simulink model "vehicle_model10DOF"  (R2020a)
settings: Solver=VariableStepAuto  StartTime=0.0  StopTime=10.0  RelTol=1e-3
values from neighbouring files (symbols this model uses):
  a = 1.05    [model_init.m]
  b = 1.8-a    (= 0.75)    [model_init.m]
  Bd = 0.1    [model_init.m]
  c = 1.5    [model_init.m]
  I = m*a*b    (= 1496.25)    [model_init.m]
  Idf = 0.805    [model_init.m]
  Idr = 0.805    [model_init.m]
  m = 1900    [model_init.m]
  r = 0.3284    [model_init.m]
undefined symbols (not defined in the file or in its folder): psi0, psidot0, vw, wfl0, wfr0, wrl0, wrr0, X0, xdot0, Y0, ydot0
settings Model: Creator=Ivona  LastModifiedBy=Ivona

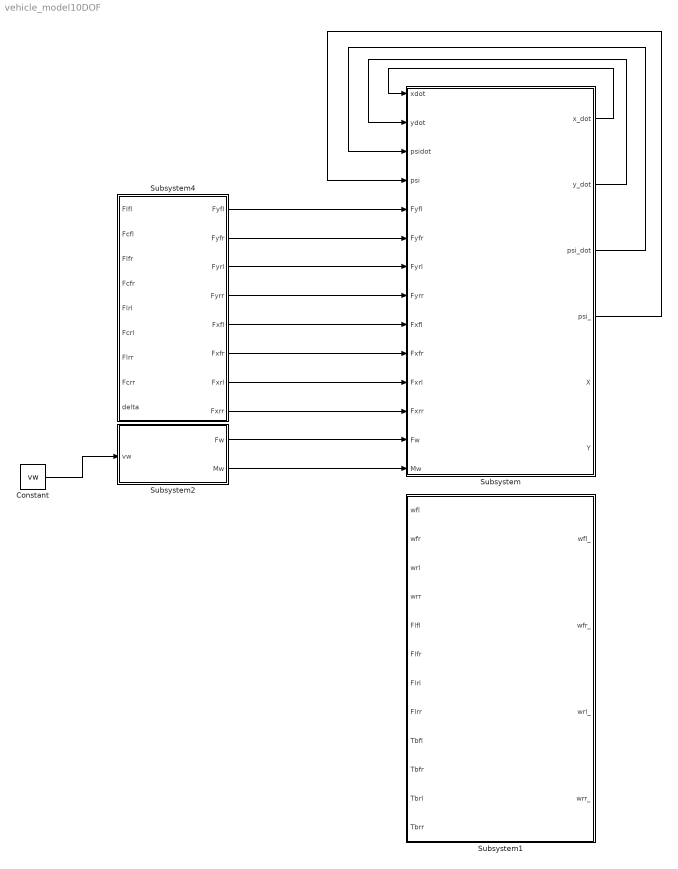
== system vehicle_model10DOF ==
  Constant : Constant  Value=vw
  Subsystem : Subsystem
  Subsystem1 : Subsystem
  Subsystem2 : Subsystem
  Subsystem4 : Subsystem
  wires:
  Subsystem/4(psi_) -> Subsystem/4(psi)
  Constant/1 -> Subsystem2/1(vw)
  Subsystem/3(psi_dot) -> Subsystem/3(psidot)
  Subsystem/2(y_dot) -> Subsystem/2(ydot)
  Subsystem4/3(Fyrl) -> Subsystem/7(Fyrl)
  Subsystem4/7(Fxrl) -> Subsystem/11(Fxrl)
  Subsystem/1(x_dot) -> Subsystem/1(xdot)
  Subsystem4/6(Fxfr) -> Subsystem/10(Fxfr)
  Subsystem4/5(Fxfl) -> Subsystem/9(Fxfl)
  Subsystem2/2(Mw) -> Subsystem/14(Mw)
  Subsystem2/1(Fw) -> Subsystem/13(Fw)
  Subsystem4/1(Fyfl) -> Subsystem/5(Fyfl)
  Subsystem4/4(Fyrr) -> Subsystem/8(Fyrr)
  Subsystem4/2(Fyfr) -> Subsystem/6(Fyfr)
  Subsystem4/8(Fxrr) -> Subsystem/12(Fxrr)

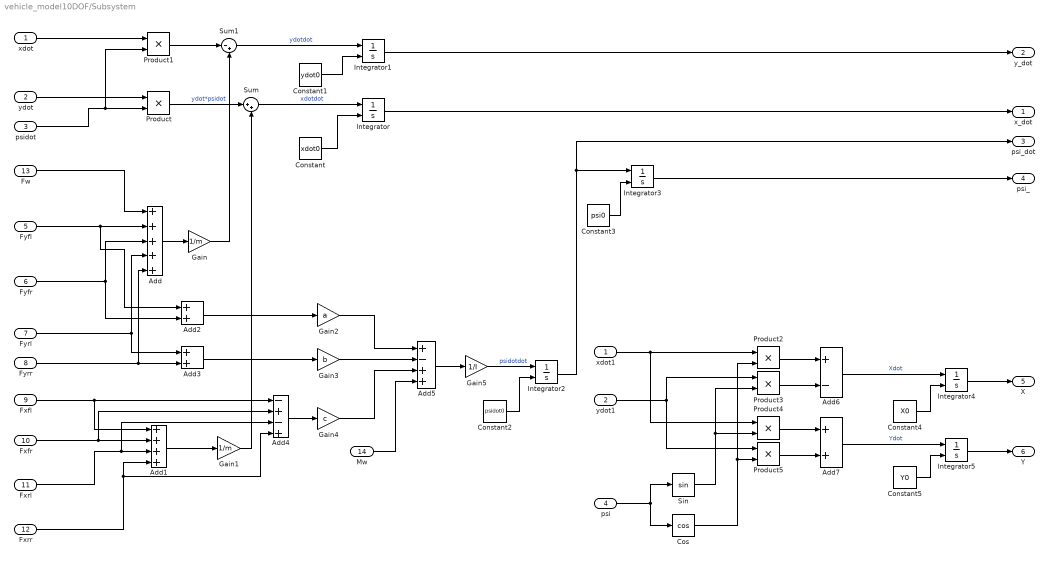
== system vehicle_model10DOF/Subsystem ==
  xdot : Inport
  ydot : Inport  Port=2
  psidot : Inport  Port=3
  psi : Inport  Port=4
  Fyfl : Inport  Port=5
  Fyfr : Inport  Port=6
  Fyrl : Inport  Port=7
  Fyrr : Inport  Port=8
  Fxfl : Inport  Port=9
  Fxfr : Inport  Port=10
  Fxrl : Inport  Port=11
  Fxrr : Inport  Port=12
  Fw : Inport  Port=13
  Mw : Inport  Port=14
  Add : Sum  Inputs=+++++
  Add1 : Sum  Inputs=++++
  Add2 : Sum
  Add3 : Sum
  Add4 : Sum  Inputs=-+-+
  Add5 : Sum  Inputs=+-++
  Add6 : Sum  Inputs=+-
  Add7 : Sum
  Constant : Constant  Value=xdot0
  Constant1 : Constant  Value=ydot0
  Constant2 : Constant  Value=psidot0
  Constant3 : Constant  Value=psi0
  Constant4 : Constant  Value=X0
  Constant5 : Constant  Value=Y0
  Cos : Trigonometry  Operator=cos
  Gain : Gain  Gain=1/m
  Gain1 : Gain  Gain=1/m
  Gain2 : Gain  Gain=a
  Gain3 : Gain  Gain=b
  Gain4 : Gain  Gain=c
  Gain5 : Gain  Gain=1/I
  Integrator{,1..5} (6 alike) : Integrator  InitialConditionSource=external
  Product{,1..5} (6 alike) : Product
  Sin : Trigonometry
  Sum : Sum  Inputs=|++
  Sum1 : Sum  Inputs=|-+
  xdot1 : InportShadow
  ydot1 : InportShadow  Port=2
  x_dot : Outport
  y_dot : Outport  Port=2
  psi_dot : Outport  Port=3
  psi_ : Outport  Port=4
  X : Outport  Port=5
  Y : Outport  Port=6
  wires:
  ydot/1 -> Product/1
  psidot/1 -> Product1/2, Product/2
  Fyfl/1 -> Add/2, Add2/1
  Fyfr/1 -> Add/3, Add2/2
  Fyrl/1 -> Add3/1, Add/4
  Fyrr/1 -> Add/5, Add3/2
  Add/1 -> Gain/1
  Product/1 -> Sum/1  "ydot*psidot"
  Sum/1 -> Integrator/1  "xdotdot"
  Constant/1 -> Integrator/2
  Integrator/1 -> x_dot/1
  xdot/1 -> Product1/1
  Product1/1 -> Sum1/1
  Fxfl/1 -> Add1/1, Add4/1
  Fxfr/1 -> Add4/2, Add1/2
  Fxrl/1 -> Add4/3, Add1/3
  Fxrr/1 -> Add4/4, Add1/4
  Add1/1 -> Gain1/1
  Sum1/1 -> Integrator1/1  "ydotdot"
  Constant1/1 -> Integrator1/2
  Integrator1/1 -> y_dot/1
  Add2/1 -> Gain2/1
  Add3/1 -> Gain3/1
  Add4/1 -> Gain4/1
  Gain2/1 -> Add5/1
  Gain3/1 -> Add5/2
  Gain4/1 -> Add5/3
  Add5/1 -> Gain5/1
  Gain5/1 -> Integrator2/1  "psidotdot"
  Constant2/1 -> Integrator2/2
  Integrator2/1 -> Integrator3/1, psi_dot/1
  Integrator3/1 -> psi_/1
  Constant3/1 -> Integrator3/2
  psi/1 -> Sin/1, Cos/1
  Product2/1 -> Add6/1
  Product3/1 -> Add6/2
  xdot1/1 -> Product4/1, Product2/1
  Cos/1 -> Product5/2, Product2/2
  ydot1/1 -> Product5/1, Product3/1
  Sin/1 -> Product4/2, Product3/2
  Product4/1 -> Add7/1
  Product5/1 -> Add7/2
  Add6/1 -> Integrator4/1  "Xdot"
  Integrator4/1 -> X/1
  Constant4/1 -> Integrator4/2
  Add7/1 -> Integrator5/1  "Ydot"
  Integrator5/1 -> Y/1
  Constant5/1 -> Integrator5/2
  Gain/1 -> Sum1/2
  Gain1/1 -> Sum/2
  Fw/1 -> Add/1
  Mw/1 -> Add5/4

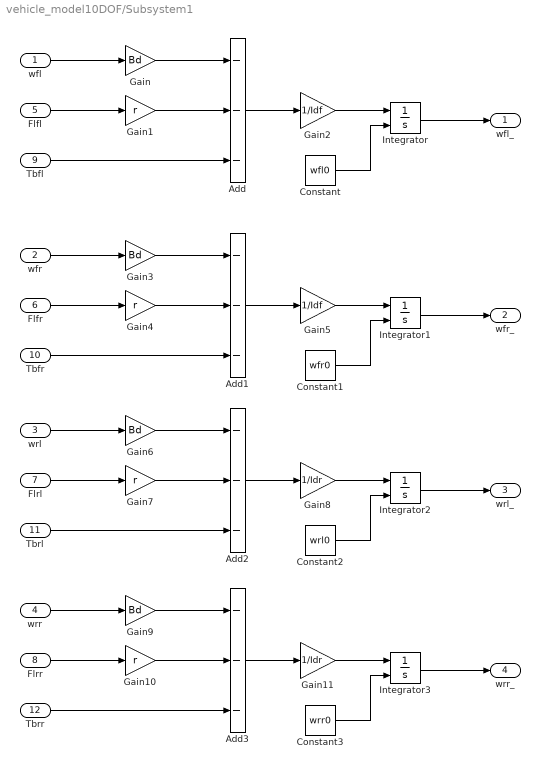
== system vehicle_model10DOF/Subsystem1 ==
  wfl : Inport
  wfr : Inport  Port=2
  wrl : Inport  Port=3
  wrr : Inport  Port=4
  Flfl : Inport  Port=5
  Flfr : Inport  Port=6
  Flrl : Inport  Port=7
  Flrr : Inport  Port=8
  Tbfl : Inport  Port=9
  Tbfr : Inport  Port=10
  Tbrl : Inport  Port=11
  Tbrr : Inport  Port=12
  Add{,1..3} (4 alike) : Sum  Inputs=---
  Constant : Constant  Value=wfl0
  Constant1 : Constant  Value=wfr0
  Constant2 : Constant  Value=wrl0
  Constant3 : Constant  Value=wrr0
  Gain{,3,6,9} (4 alike) : Gain  Gain=Bd
  Gain{1,4,7,10} (4 alike) : Gain  Gain=r
  Gain11 : Gain  Gain=1/Idr
  Gain2 : Gain  Gain=1/Idf
  Gain5 : Gain  Gain=1/Idf
  Gain8 : Gain  Gain=1/Idr
  Integrator{,1..3} (4 alike) : Integrator  InitialConditionSource=external
  wfl_ : Outport
  wfr_ : Outport  Port=2
  wrl_ : Outport  Port=3
  wrr_ : Outport  Port=4
  wires:
  Gain/1 -> Add/1
  Tbfl/1 -> Add/3
  Flfl/1 -> Gain1/1
  wfl/1 -> Gain/1
  Gain1/1 -> Add/2
  Add/1 -> Gain2/1
  Gain2/1 -> Integrator/1
  Constant/1 -> Integrator/2
  Integrator/1 -> wfl_/1
  Tbfr/1 -> Add1/3
  wfr/1 -> Gain3/1
  Gain3/1 -> Add1/1
  Flfr/1 -> Gain4/1
  Gain4/1 -> Add1/2
  Add1/1 -> Gain5/1
  Integrator1/1 -> wfr_/1
  Gain5/1 -> Integrator1/1
  Constant1/1 -> Integrator1/2
  Gain8/1 -> Integrator2/1
  Add2/1 -> Gain8/1
  Tbrl/1 -> Add2/3
  wrl/1 -> Gain6/1
  Constant2/1 -> Integrator2/2
  Integrator2/1 -> wrl_/1
  Gain7/1 -> Add2/2
  Gain6/1 -> Add2/1
  Flrl/1 -> Gain7/1
  Gain11/1 -> Integrator3/1
  Add3/1 -> Gain11/1
  Tbrr/1 -> Add3/3
  wrr/1 -> Gain9/1
  Constant3/1 -> Integrator3/2
  Integrator3/1 -> wrr_/1
  Gain10/1 -> Add3/2
  Gain9/1 -> Add3/1
  Flrr/1 -> Gain10/1

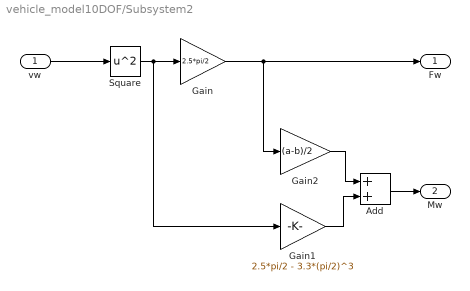
== system vehicle_model10DOF/Subsystem2 ==
  vw : Inport
  Add : Sum
  Gain : Gain  Gain=2.5*pi/2
  Gain1 : Gain  Gain=2.5*pi/2 - 3.3*(pi/2)^3
  Gain2 : Gain  Gain=(a-b)/2
  Square : Math  Operator=square  SaturateOnIntegerOverflow=on
  Fw : Outport
  Mw : Outport  Port=2
  wires:
  vw/1 -> Square/1
  Square/1 -> Gain1/1, Gain/1
  Gain/1 -> Gain2/1, Fw/1
  Gain2/1 -> Add/1
  Gain1/1 -> Add/2
  Add/1 -> Mw/1

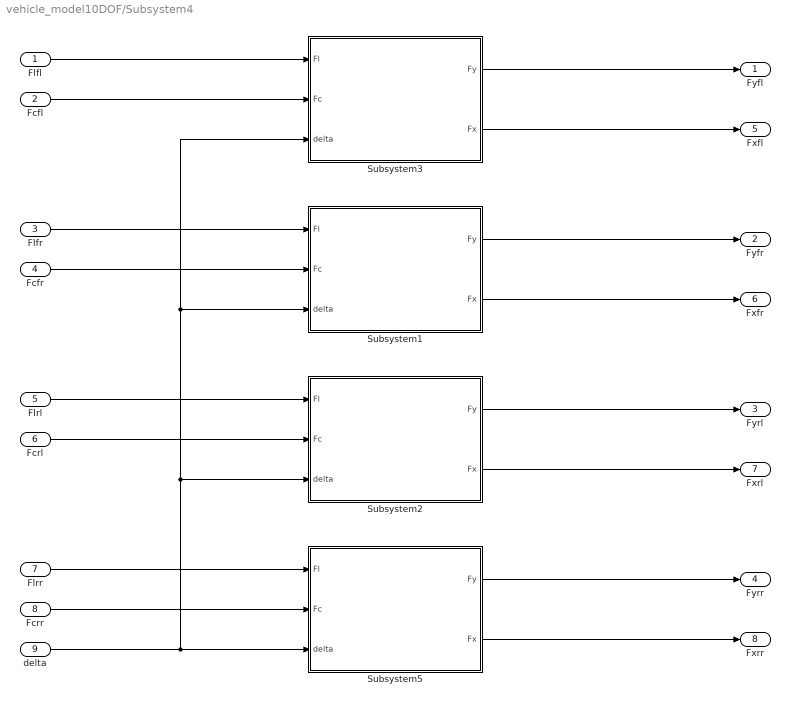
== system vehicle_model10DOF/Subsystem4 ==
  Flfl : Inport
  Fcfl : Inport  Port=2
  Flfr : Inport  Port=3
  Fcfr : Inport  Port=4
  Flrl : Inport  Port=5
  Fcrl : Inport  Port=6
  Flrr : Inport  Port=7
  Fcrr : Inport  Port=8
  delta : Inport  Port=9
  Subsystem1 : Subsystem
  Subsystem2 : Subsystem
  Subsystem3 : Subsystem
  Subsystem5 : Subsystem
  Fyfl : Outport
  Fyfr : Outport  Port=2
  Fyrl : Outport  Port=3
  Fyrr : Outport  Port=4
  Fxfl : Outport  Port=5
  Fxfr : Outport  Port=6
  Fxrl : Outport  Port=7
  Fxrr : Outport  Port=8
  wires:
  Flfl/1 -> Subsystem3/1(Fl)
  Fcfl/1 -> Subsystem3/2(Fc)
  delta/1 -> Subsystem5/3(delta), Subsystem2/3(delta), Subsystem1/3(delta), Subsystem3/3(delta)
  Subsystem3/1(Fy) -> Fyfl/1
  Subsystem3/2(Fx) -> Fxfl/1
  Flfr/1 -> Subsystem1/1(Fl)
  Fcfr/1 -> Subsystem1/2(Fc)
  Subsystem1/1(Fy) -> Fyfr/1
  Subsystem1/2(Fx) -> Fxfr/1
  Fcrl/1 -> Subsystem2/2(Fc)
  Flrl/1 -> Subsystem2/1(Fl)
  Subsystem2/2(Fx) -> Fxrl/1
  Subsystem2/1(Fy) -> Fyrl/1
  Fcrr/1 -> Subsystem5/2(Fc)
  Flrr/1 -> Subsystem5/1(Fl)
  Subsystem5/2(Fx) -> Fxrr/1
  Subsystem5/1(Fy) -> Fyrr/1

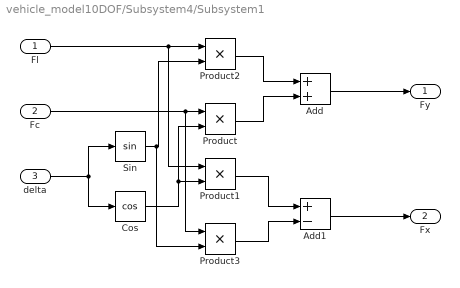
== system vehicle_model10DOF/Subsystem4/Subsystem1 ==
  Fl : Inport
  Fc : Inport  Port=2
  delta : Inport  Port=3
  Add : Sum
  Add1 : Sum  Inputs=+-
  Cos : Trigonometry  Operator=cos
  Product{,1..3} (4 alike) : Product
  Sin : Trigonometry
  Fy : Outport
  Fx : Outport  Port=2
  wires:
  Add1/1 -> Fx/1
  Product3/1 -> Add1/2
  Product1/1 -> Add1/1
  Add/1 -> Fy/1
  Product/1 -> Add/2
  Product2/1 -> Add/1
  Cos/1 -> Product/2, Product1/2
  Fc/1 -> Product/1, Product3/1
  Sin/1 -> Product2/2, Product3/2
  Fl/1 -> Product2/1, Product1/1
  delta/1 -> Sin/1, Cos/1

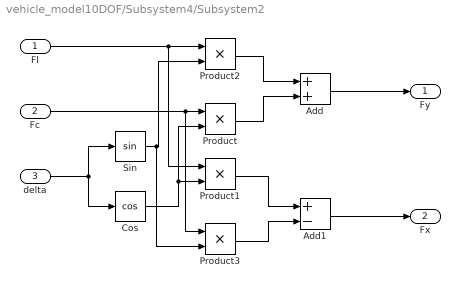
== system vehicle_model10DOF/Subsystem4/Subsystem2 ==
  Fl : Inport
  Fc : Inport  Port=2
  delta : Inport  Port=3
  Add : Sum
  Add1 : Sum  Inputs=+-
  Cos : Trigonometry  Operator=cos
  Product{,1..3} (4 alike) : Product
  Sin : Trigonometry
  Fy : Outport
  Fx : Outport  Port=2
  wires:
  delta/1 -> Cos/1, Sin/1
  Fl/1 -> Product1/1, Product2/1
  Sin/1 -> Product3/2, Product2/2
  Fc/1 -> Product3/1, Product/1
  Cos/1 -> Product1/2, Product/2
  Product2/1 -> Add/1
  Product/1 -> Add/2
  Add/1 -> Fy/1
  Product1/1 -> Add1/1
  Product3/1 -> Add1/2
  Add1/1 -> Fx/1

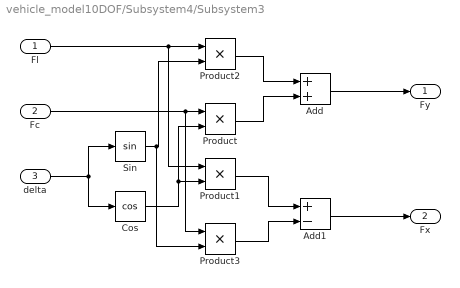
== system vehicle_model10DOF/Subsystem4/Subsystem3 ==
  Fl : Inport
  Fc : Inport  Port=2
  delta : Inport  Port=3
  Add : Sum
  Add1 : Sum  Inputs=+-
  Cos : Trigonometry  Operator=cos
  Product{,1..3} (4 alike) : Product
  Sin : Trigonometry
  Fy : Outport
  Fx : Outport  Port=2
  wires:
  delta/1 -> Cos/1, Sin/1
  Fl/1 -> Product1/1, Product2/1
  Sin/1 -> Product3/2, Product2/2
  Fc/1 -> Product3/1, Product/1
  Cos/1 -> Product1/2, Product/2
  Product2/1 -> Add/1
  Product/1 -> Add/2
  Add/1 -> Fy/1
  Product1/1 -> Add1/1
  Product3/1 -> Add1/2
  Add1/1 -> Fx/1

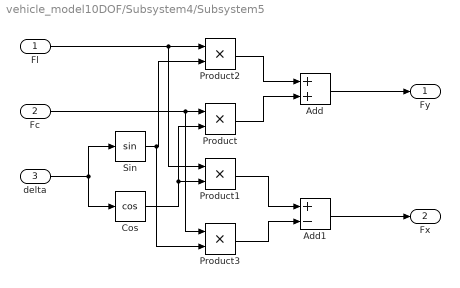
== system vehicle_model10DOF/Subsystem4/Subsystem5 ==
  Fl : Inport
  Fc : Inport  Port=2
  delta : Inport  Port=3
  Add : Sum
  Add1 : Sum  Inputs=+-
  Cos : Trigonometry  Operator=cos
  Product{,1..3} (4 alike) : Product
  Sin : Trigonometry
  Fy : Outport
  Fx : Outport  Port=2
  wires:
  delta/1 -> Cos/1, Sin/1
  Fl/1 -> Product1/1, Product2/1
  Sin/1 -> Product3/2, Product2/2
  Fc/1 -> Product3/1, Product/1
  Cos/1 -> Product1/2, Product/2
  Product2/1 -> Add/1
  Product/1 -> Add/2
  Add/1 -> Fy/1
  Product1/1 -> Add1/1
  Product3/1 -> Add1/2
  Add1/1 -> Fx/1
